simulink model "Tire1_basic00"  (R2022a)
settings: Solver=VariableStepAuto  StartTime=0.0  StopTime=100  RelTol=1e-3
values from neighbouring files (symbols this model uses):
  Tire_MagicB = 10    [TireParam.m]
  Tire_MagicC = 1.9    [TireParam.m]
  Tire_MagicD = 0.9    [TireParam.m]
  Tire_MagicE = 0.97    [TireParam.m]
libraries: fl_lib x4, nesl_utility x4, simulink x1, sdl_lib x1
settings Model: Creator=amyyang  LastModifiedBy=amyyang
settings SolverCC: AlgebraicLoopSolver=TrustRegion
settings DebuggingCC: UnconnectedInputMsg=warning  UnconnectedOutputMsg=warning  UnconnectedLineMsg=warning  SFMachineParentedDataDiag=warning
settings RTWCC: DLArmComputeVersion=19.05
settings SimscapeCC: SimscapeLogType=local  SimscapeLogToSDI=on  SimscapeLogLimitData=off

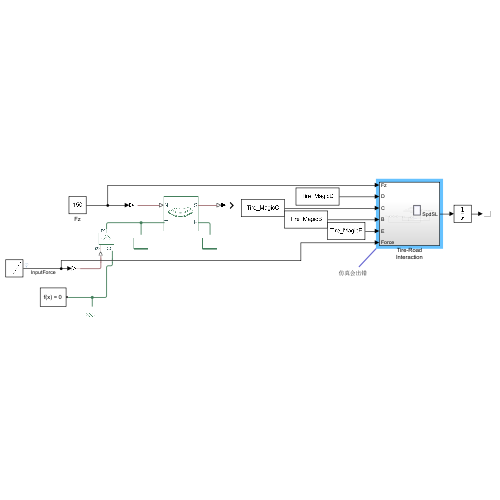
[thumbnail: Simulink's stored preview of the top-level diagram]
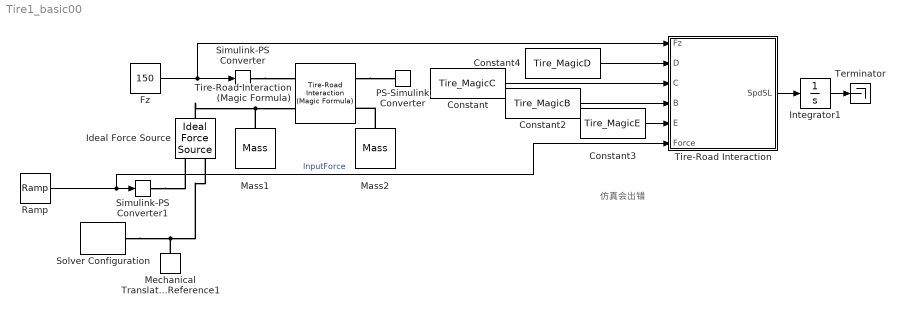
== system Tire1_basic00 ==
  note: 仿真会出错
  Constant : Constant  Value=Tire_MagicC
  Constant2 : Constant  Value=Tire_MagicB
  Constant3 : Constant  Value=Tire_MagicE
  Constant4 : Constant  Value=Tire_MagicD
  Fz : Constant  Value=150
  Ideal Force Source : fl_lib/Mechanical/Mechanical Sources/Ideal Force Source
      settings: SourceProductBaseCode=PW,SS,VE
  Integrator1 : Integrator
  Mass1 : fl_lib/Mechanical/Translational Elements/Mass  mass=1 kg  num_ports=foundation.enum.numPorts2.one  v_specify=off  v_priority=High  v=0 m/s  v_nominal_specify=off  v_nominal_unit=m/s  v_nominal_value=1  f_specify=off  f_priority=None  f=0 N  f_nominal_specify=off  f_nominal_unit=N  f_nominal_value=1
      settings: SourceProductBaseCode=PW,SS,VE
  Mass2 : fl_lib/Mechanical/Translational Elements/Mass  mass=50 kg  num_ports=foundation.enum.numPorts2.one  v_specify=off  v_priority=High  v=0 m/s  v_nominal_specify=off  v_nominal_unit=m/s  v_nominal_value=1  f_specify=off  f_priority=None  f=0 N  f_nominal_specify=off  f_nominal_unit=N  f_nominal_value=1
      settings: SourceProductBaseCode=PW,SS,VE  LogSimulationData=on
  Mechanical Translational Reference1 : fl_lib/Mechanical/Translational Elements/Mechanical Translational Reference
      settings: SourceProductBaseCode=PW,SS,VE
  PS-Simulink Converter : nesl_utility/PS-Simulink Converter  PhysicalDomain=network_engine_domain  SubClassName=ps_output  LeftPortType=input  RightPortType=output  PseudoPeriodic=off  Frequencies=[]  VectorFormat=1-D array  Unit=inherit  AffineConversion=off
      settings: SourceProductBaseCode=SS,PW,VE
  Ramp : simulink/Sources/Ramp  slope=10  start=0  InitialOutput=0
  Simulink-PS Converter : nesl_utility/Simulink-PS Converter  PhysicalDomain=network_engine_domain  SubClassName=ps_input  LeftPortType=input  RightPortType=output  PseudoPeriodic=off  Frequencies=[]  NoiseDistribution=none  NoiseParameters=[]  Unit=1  AffineConversion=off  FilteringAndDerivatives=provide  SimscapeFilterOrder=1  InputFilterTimeConstant=0.001  UdotUserProvided=0
      settings: SourceProductBaseCode=SS,PW,VE
  Simulink-PS Converter1 : nesl_utility/Simulink-PS Converter  PhysicalDomain=network_engine_domain  SubClassName=ps_input  LeftPortType=input  RightPortType=output  PseudoPeriodic=off  Frequencies=[]  NoiseDistribution=none  NoiseParameters=[]  Unit=1  AffineConversion=off  FilteringAndDerivatives=provide  SimscapeFilterOrder=1  InputFilterTimeConstant=0.001  UdotUserProvided=0
      settings: SourceProductBaseCode=SS,PW,VE
  Solver Configuration : nesl_utility/Solver Configuration  PhysicalDomain=network_engine_domain  SubClassName=solver  LeftPortType=input  RightPortType=generic  Tones=[]  Harmonics=[]  SimulateNoise=off  Profile=off  UseLocalSampling=off  EnableSwitchedLinearOptims=on  FrequencyDomain=off  UseCCode=off  RelTol=0.001  AbsTol=1e-06  MinStep=1e-09  ToWorkspace=off  RevertToSquareIcSolve=off  NumHomotopyIterations=100  PhasorMode=off  PhasorModeNumHarmonics=1  IndexReductionMethod=DerivativeReplacement  DoDC=off  ResidualTolerance=1e-09  UseLocalSolver=off  LocalSolverChoice=NE_BACKWARD_EULER_ADVANCER  LocalSolverSampleTime=0.001  DoFixedCost=off  MaxNonlinIter=3  MaxModeIter=2  ComputeImpulses=off  ImpulseIterations=2  LinearAlgebra=auto  LinearAlgebraNumThread=0  EquationFormulation=NE_TIME_EF  DelaysMemoryBudget=1024  AutomaticFiltering=on  FilteringTimeConstant=0.001  PartitionStorageMethod=AS_NEEDED  PartitionMemoryBudget=1024  PartitionMethod=ROBUST
      settings: SourceProductBaseCode=SS,PW,VE
  Terminator : Terminator
  Tire-Road Interaction : Subsystem
  Tire-Road Interaction (Magic Formula) : sdl_lib/Tires & Vehicles/Tire Subcomponents/Tire-Road Interaction (Magic Formula)  parameterization=sdl.enum.magic_tire_model.constant  F_z1=3000 N  F_x1=3500 N  kappa1=10  B_m=Tire_MagicB  C_m=Tire_MagicC  D_m=Tire_MagicD  E_m=Tire_MagicE  fz0=4000 N  p_Cx=1.685  p_Dx=[1.21, -.037]  p_Ex=[.344, .095, -.02, 0]  p_Kx=[21.51, -.163, .245]  p_Hx=[-.002, .002]  p_Vx=[0, 0]  v_tr_thr=0.1 m/s
      settings: SourceProductBaseCode=LD  LogSimulationData=on  InternalSimscapePortConfiguration="{\"Bottom\":[],\"Left\":[{\"id\":\"N\",\"label\":\"N\",\"type\":\"input\"},{\"id\":\"T\",\"label\":\"T\",\"type\":\"foundation.mechanical.translational.translational\"}],\"Right\":[{\"id\":\"S\",\"label\":\"S\",\"type\":\"output\"},{\"id\":\"H\",\"label\":\"H\",\"type\":\"foundation.mechanical.translational.translational\"}],\"Top\":[]}"
  wires:
  Fz/1 -> Tire-Road Interaction/1(Fz), Simulink-PS Converter/1
  Integrator1/1 -> Terminator/1
  Constant4/1 -> Tire-Road Interaction/2(D)
  Constant/1 -> Tire-Road Interaction/3(C)
  Constant2/1 -> Tire-Road Interaction/4(B)
  Constant3/1 -> Tire-Road Interaction/5(E)
  Ramp/1 -> Tire-Road Interaction/6(Force), Simulink-PS Converter1/1  "InputForce"
  Tire-Road Interaction/1(SpdSL) -> Integrator1/1
  connections:
  Ideal Force Source/LConn1 -- Mass1/LConn1 -- Tire-Road Interaction (Magic Formula)/LConn2
  Simulink-PS Converter/RConn1 -- Tire-Road Interaction (Magic Formula)/LConn1
  Mechanical Translational Reference1/LConn1 -- Solver Configuration/RConn1 -- Ideal Force Source/RConn2
  Simulink-PS Converter1/RConn1 -- Ideal Force Source/RConn1
  Tire-Road Interaction (Magic Formula)/RConn1 -- PS-Simulink Converter/LConn1
  Mass2/LConn1 -- Tire-Road Interaction (Magic Formula)/RConn2

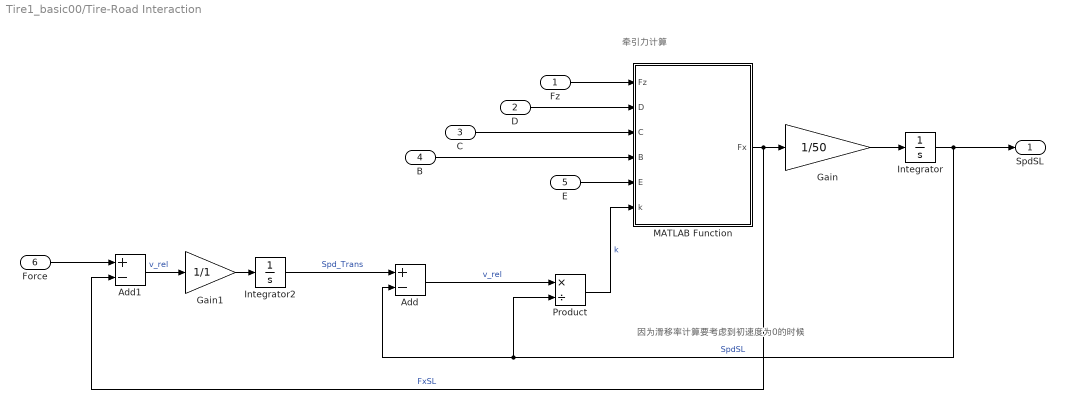
== system Tire1_basic00/Tire-Road Interaction ==
  note: 因为滑移率计算要考虑到初速度为0的时候
  note: 牵引力计算
  Fz : Inport
  D : Inport  Port=2
  C : Inport  Port=3
  B : Inport  Port=4
  E : Inport  Port=5
  Force : Inport  Port=6
  Add : Sum  Inputs=+-
  Add1 : Sum  Inputs=+-
  Gain : Gain  Gain=1/50
  Gain1 : Gain  Gain=1/1
  Integrator : Integrator
  Integrator2 : Integrator
  MATLAB Function : MATLAB Function  TreatAsAtomicUnit=on
  Product : Product  Inputs=*/
  SpdSL : Outport
  wires:
  D/1 -> MATLAB Function/2(D)
  Add1/1 -> Gain1/1  "v_rel"
  Integrator/1 -> SpdSL/1, Add/2, Product/2  "SpdSL"
  Product/1 -> MATLAB Function/6(k)  "k"
  MATLAB Function/1(Fx) -> Add1/2, Gain/1  "FxSL"
  Gain1/1 -> Integrator2/1
  Add/1 -> Product/1  "v_rel"
  Force/1 -> Add1/1
  Gain/1 -> Integrator/1
  Integrator2/1 -> Add/1  "Spd_Trans"
  Fz/1 -> MATLAB Function/1(Fz)
  E/1 -> MATLAB Function/5(E)
  B/1 -> MATLAB Function/4(B)
  C/1 -> MATLAB Function/3(C)

== matlab function Tire1_basic00/Tire-Road Interaction/MATLAB Function ==
  data: Fz input; D input; C input; B input; E input; Fx output; k input
function Fx = fcn(Fz,D,C,B,E,k)

Fx = Fz * D*sin(C*atan(B*k - E*(B*k - atan(B*k))));
end
